simulink model "vehicle5"  (R2017a)
settings: Solver=VariableStepAuto  StartTime=0.0  StopTime=10.0  RelTol=1e-3
undefined symbols (not defined in the file or in its folder): magnitude
libraries: elvio x10
settings Model: Creator=tstef  LastModifiedBy=tstef

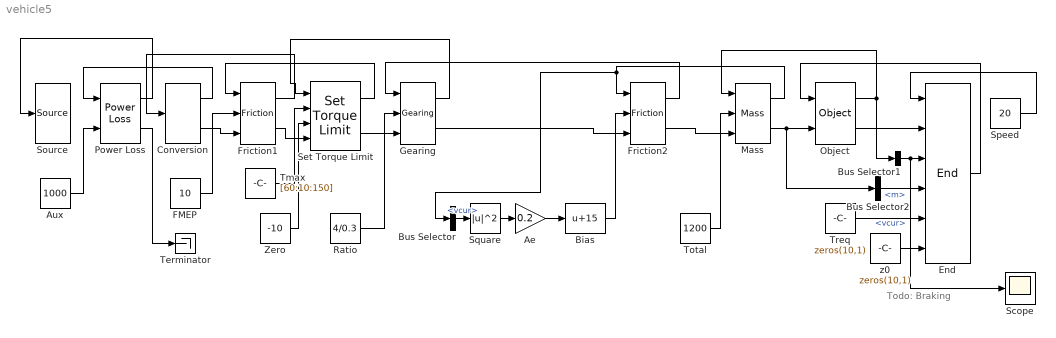
== system vehicle5 ==
  note: Todo: Braking
  Ae : Gain  Gain=0.2
  Aux : Constant  Value=1000
  Bias : Bias  Bias=15
  Bus Selector : BusSelector  OutputSignals=vcur
  Bus Selector1 : BusSelector  OutputSignals=vcur
  Bus Selector2 : BusSelector  OutputSignals=m
  Conversion : elvio/Basics/Conversion
  End : elvio/Basics/End
  FMEP : Constant  Value=10
  Friction1 : elvio/Basics/Friction
  Friction2 : elvio/Basics/Friction
  Gearing : elvio/Basics/Gearing
  Mass : elvio/Basics/Mass
  Object : elvio/Basics/Object
  Power Loss : elvio/Basics/Power Loss
  Ratio : Constant  Value=4/0.3
  Scope : Scope
  Set Torque Limit : elvio/Basics/Set Torque Limit
  Source : elvio/Basics/Source
  Speed : Constant  Value=20
  Square : Math  Operator=magnitude^2  SaturateOnIntegerOverflow=on
  Terminator : Terminator
  Tmax : Constant  Value=[60:10:150]
  Total : Constant  Value=1200
  Treq : Constant  Value=zeros(10,1)
  Zero : Constant  Value=-10
  z0 : Constant  Value=zeros(10,1)
  wires:
  Friction2/2 -> Mass/3
  Gearing/2 -> Friction2/3
  Set Torque Limit/2 -> Gearing/3
  Friction1/2 -> Set Torque Limit/4
  Conversion/2 -> Friction1/3
  Power Loss/1 -> Source/1
  Speed/1 -> End/1
  Conversion/1 -> Power Loss/1
  Friction1/1 -> Conversion/1
  Set Torque Limit/1 -> Friction1/1
  Gearing/1 -> Set Torque Limit/1
  Friction2/1 -> Gearing/1
  Mass/1 -> Friction2/1, Bus Selector/1
  Object/1 -> Mass/1, Bus Selector1/1
  End/1 -> Object/1
  FMEP/1 -> Friction1/2
  Aux/1 -> Power Loss/2
  Tmax/1 -> Set Torque Limit/2
  Zero/1 -> Set Torque Limit/3
  Ratio/1 -> Gearing/2
  Total/1 -> Mass/2
  Object/2 -> End/2
  Power Loss/2 -> Terminator/1
  Square/1 -> Ae/1
  Ae/1 -> Bias/1
  Bias/1 -> Friction2/2
  Bus Selector/1 -> Square/1  "<vcur>"
  Bus Selector1/1 -> Scope/1, End/3  "<vcur>"
  Mass/2 -> Bus Selector2/1, Object/2
  z0/1 -> End/6
  Treq/1 -> End/5
  Bus Selector2/1 -> End/4  "<m>"
